simulink model "TEP_Final_NoScript"  (R2024a)
settings: Solver=FixedStepAuto  StartTime=0.0  StopTime=10  FixedStep=1/3600  RelTol=1e-3
model workspace (MAT data in the model file):
  AD : Simulink.Parameter (value not decoded)
  AG : Simulink.Parameter (value not decoded)
  AH : Simulink.Parameter (value not decoded)
  AV : Simulink.Parameter (value not decoded)
  AVP : Simulink.Parameter (value not decoded)
  BCHL : Simulink.Parameter (value not decoded)
  BCHV : Simulink.Parameter (value not decoded)
  BD : Simulink.Parameter (value not decoded)
  BG : Simulink.Parameter (value not decoded)
  BH : Simulink.Parameter (value not decoded)
  BVP : Simulink.Parameter (value not decoded)
  CD : Simulink.Parameter (value not decoded)
  CG : Simulink.Parameter (value not decoded)
  CH : Simulink.Parameter (value not decoded)
  CVP : Simulink.Parameter (value not decoded)
  XMW : Simulink.Parameter (value not decoded)
  XNS : Simulink.Parameter (value not decoded)
  XNSE : Simulink.Parameter (value not decoded)
symbols that are objects in the model workspace (value not decoded): AD, AG, AH, AV, AVP, BD, BG, BH, BVP, CD, CG, CH, CVP, XMW, XNS, XNSE
undefined symbols (not defined in the file or in its folder): magnitude, msgbox, SETPT, XMEAS, XMV
libraries: mylib x360, dspindex x28
(part 14 of 14)

== system TEP_Final_NoScript/Random number generator1/Stream Measurements SMEAS Gas analysis/If Action Subsystem3/Subsystem/Stream 9/Subsystem/TESUB6 XMNSED ==
  G : Inport
  Process Noise I=1-12 G New : mylib/Process Noise I=1-12 G New  SystemSampleTime=-1  VariantActivationTime=update diagram  AllowFlexibleInterface=on  Latency=0  AutoFrameSizeCalculation=off
      settings: SourceProductName=TEP Library
  XNSED : Constant  Value=0.1
  XMNSED : Outport  VectorParamsAs1DForOutWhenUnconnected=off
  G_NEW : Outport  Port=2  VectorParamsAs1DForOutWhenUnconnected=off
  wires:
  XNSED/1 -> Process Noise I=1-12 G New/1
  Process Noise I=1-12 G New/1 -> XMNSED/1
  G/1 -> Process Noise I=1-12 G New/2
  Process Noise I=1-12 G New/2 -> G_NEW/1

== system TEP_Final_NoScript/Random number generator1/Stream Measurements SMEAS Gas analysis/If Action Subsystem3/Subsystem/Stream 9/Subsystem/TESUB6 XMNSEE ==
  G : Inport
  Process Noise I=1-12 G New : mylib/Process Noise I=1-12 G New  SystemSampleTime=-1  VariantActivationTime=update diagram  AllowFlexibleInterface=on  Latency=0  AutoFrameSizeCalculation=off
      settings: SourceProductName=TEP Library
  XNSEE : Constant  Value=0.25
  XMNSEE : Outport  VectorParamsAs1DForOutWhenUnconnected=off
  G_NEW : Outport  Port=2  VectorParamsAs1DForOutWhenUnconnected=off
  wires:
  XNSEE/1 -> Process Noise I=1-12 G New/1
  Process Noise I=1-12 G New/1 -> XMNSEE/1
  G/1 -> Process Noise I=1-12 G New/2
  Process Noise I=1-12 G New/2 -> G_NEW/1

== system TEP_Final_NoScript/Random number generator1/Stream Measurements SMEAS Gas analysis/If Action Subsystem3/Subsystem/Stream 9/Subsystem/TESUB6 XMNSEF ==
  G : Inport
  Process Noise I=1-12 G New : mylib/Process Noise I=1-12 G New  SystemSampleTime=-1  VariantActivationTime=update diagram  AllowFlexibleInterface=on  Latency=0  AutoFrameSizeCalculation=off
      settings: SourceProductName=TEP Library
  XNSEF : Constant  Value=0.025
  XMNSEF : Outport  VectorParamsAs1DForOutWhenUnconnected=off
  G_NEW : Outport  Port=2  VectorParamsAs1DForOutWhenUnconnected=off
  wires:
  XNSEF/1 -> Process Noise I=1-12 G New/1
  Process Noise I=1-12 G New/1 -> XMNSEF/1
  G/1 -> Process Noise I=1-12 G New/2
  Process Noise I=1-12 G New/2 -> G_NEW/1

== system TEP_Final_NoScript/Random number generator1/Stream Measurements SMEAS Gas analysis/If Action Subsystem3/Subsystem/Stream 9/Subsystem/TESUB6 XMNSEG ==
  G : Inport
  Process Noise I=1-12 G New : mylib/Process Noise I=1-12 G New  SystemSampleTime=-1  VariantActivationTime=update diagram  AllowFlexibleInterface=on  Latency=0  AutoFrameSizeCalculation=off
      settings: SourceProductName=TEP Library
  XNSEG : Constant  Value=0.05
  XMNSEG : Outport  VectorParamsAs1DForOutWhenUnconnected=off
  G_NEW : Outport  Port=2  VectorParamsAs1DForOutWhenUnconnected=off
  wires:
  XNSEG/1 -> Process Noise I=1-12 G New/1
  Process Noise I=1-12 G New/1 -> XMNSEG/1
  G/1 -> Process Noise I=1-12 G New/2
  Process Noise I=1-12 G New/2 -> G_NEW/1

== system TEP_Final_NoScript/Random number generator1/Stream Measurements SMEAS Gas analysis/If Action Subsystem3/Subsystem/Stream 9/Subsystem/TESUB6 XMNSEH ==
  G : Inport
  Process Noise I=1-12 G New : mylib/Process Noise I=1-12 G New  SystemSampleTime=-1  VariantActivationTime=update diagram  AllowFlexibleInterface=on  Latency=0  AutoFrameSizeCalculation=off
      settings: SourceProductName=TEP Library
  XNSEH : Constant  Value=0.05
  XMNSEH : Outport  VectorParamsAs1DForOutWhenUnconnected=off
  G_NEW : Outport  Port=2  VectorParamsAs1DForOutWhenUnconnected=off
  wires:
  XNSEH/1 -> Process Noise I=1-12 G New/1
  Process Noise I=1-12 G New/1 -> XMNSEH/1
  G/1 -> Process Noise I=1-12 G New/2
  Process Noise I=1-12 G New/2 -> G_NEW/1

== system TEP_Final_NoScript/Random number generator1/Stream Measurements SMEAS Product analysis/If Action Subsystem3/Subsystem/Subsystem1/Subsystem/TESUB6 XMNSED ==
  G : Inport
  Process Noise I=1-12 G New : mylib/Process Noise I=1-12 G New  SystemSampleTime=-1  VariantActivationTime=update diagram  AllowFlexibleInterface=on  Latency=0  AutoFrameSizeCalculation=off
      settings: SourceProductName=TEP Library
  XNS(37) : Constant  Value=0.01
  XMNS : Outport  VectorParamsAs1DForOutWhenUnconnected=off
  G_NEW : Outport  Port=2  VectorParamsAs1DForOutWhenUnconnected=off
  wires:
  XNS(37)/1 -> Process Noise I=1-12 G New/1
  Process Noise I=1-12 G New/1 -> XMNS/1
  G/1 -> Process Noise I=1-12 G New/2
  Process Noise I=1-12 G New/2 -> G_NEW/1

== system TEP_Final_NoScript/Random number generator1/Stream Measurements SMEAS Product analysis/If Action Subsystem3/Subsystem/Subsystem1/Subsystem/TESUB6 XMNSEE ==
  G : Inport
  Process Noise I=1-12 G New : mylib/Process Noise I=1-12 G New  SystemSampleTime=-1  VariantActivationTime=update diagram  AllowFlexibleInterface=on  Latency=0  AutoFrameSizeCalculation=off
      settings: SourceProductName=TEP Library
  XNS(38) : Constant  Value=0.01
  XMNS : Outport  VectorParamsAs1DForOutWhenUnconnected=off
  G_NEW : Outport  Port=2  VectorParamsAs1DForOutWhenUnconnected=off
  wires:
  XNS(38)/1 -> Process Noise I=1-12 G New/1
  Process Noise I=1-12 G New/1 -> XMNS/1
  G/1 -> Process Noise I=1-12 G New/2
  Process Noise I=1-12 G New/2 -> G_NEW/1

== system TEP_Final_NoScript/Random number generator1/Stream Measurements SMEAS Product analysis/If Action Subsystem3/Subsystem/Subsystem1/Subsystem/TESUB6 XMNSEF ==
  G : Inport
  Process Noise I=1-12 G New : mylib/Process Noise I=1-12 G New  SystemSampleTime=-1  VariantActivationTime=update diagram  AllowFlexibleInterface=on  Latency=0  AutoFrameSizeCalculation=off
      settings: SourceProductName=TEP Library
  XNS(39) : Constant  Value=0.01
  XMNS : Outport  VectorParamsAs1DForOutWhenUnconnected=off
  G_NEW : Outport  Port=2  VectorParamsAs1DForOutWhenUnconnected=off
  wires:
  XNS(39)/1 -> Process Noise I=1-12 G New/1
  Process Noise I=1-12 G New/1 -> XMNS/1
  G/1 -> Process Noise I=1-12 G New/2
  Process Noise I=1-12 G New/2 -> G_NEW/1

== system TEP_Final_NoScript/Random number generator1/Stream Measurements SMEAS Product analysis/If Action Subsystem3/Subsystem/Subsystem1/Subsystem/TESUB6 XMNSEG ==
  G : Inport
  Process Noise I=1-12 G New : mylib/Process Noise I=1-12 G New  SystemSampleTime=-1  VariantActivationTime=update diagram  AllowFlexibleInterface=on  Latency=0  AutoFrameSizeCalculation=off
      settings: SourceProductName=TEP Library
  XNS(40) : Constant  Value=0.5
  XMNS : Outport  VectorParamsAs1DForOutWhenUnconnected=off
  G_NEW : Outport  Port=2  VectorParamsAs1DForOutWhenUnconnected=off
  wires:
  XNS(40)/1 -> Process Noise I=1-12 G New/1
  Process Noise I=1-12 G New/1 -> XMNS/1
  G/1 -> Process Noise I=1-12 G New/2
  Process Noise I=1-12 G New/2 -> G_NEW/1

== system TEP_Final_NoScript/Random number generator1/Stream Measurements SMEAS Product analysis/If Action Subsystem3/Subsystem/Subsystem1/Subsystem/TESUB6 XMNSEH ==
  G : Inport
  Process Noise I=1-12 G New : mylib/Process Noise I=1-12 G New  SystemSampleTime=-1  VariantActivationTime=update diagram  AllowFlexibleInterface=on  Latency=0  AutoFrameSizeCalculation=off
      settings: SourceProductName=TEP Library
  XNS(41) : Constant  Value=0.5
  XMNS : Outport  VectorParamsAs1DForOutWhenUnconnected=off
  G_NEW : Outport  Port=2  VectorParamsAs1DForOutWhenUnconnected=off
  wires:
  XNS(41)/1 -> Process Noise I=1-12 G New/1
  Process Noise I=1-12 G New/1 -> XMNS/1
  G/1 -> Process Noise I=1-12 G New/2
  Process Noise I=1-12 G New/2 -> G_NEW/1

== system TEP_Final_NoScript/Random number generator1/Stream Measurements SMEAS Product analysis/If Action Subsystem3/Subsystem/Subsystem2/Subsystem/TESUB6 XMNSED ==
  G : Inport
  Process Noise I=1-12 G New : mylib/Process Noise I=1-12 G New  SystemSampleTime=-1  VariantActivationTime=update diagram  AllowFlexibleInterface=on  Latency=0  AutoFrameSizeCalculation=off
      settings: SourceProductName=TEP Library
  XNS(37) : Constant  Value=0.01
  XMNS : Outport  VectorParamsAs1DForOutWhenUnconnected=off
  G_NEW : Outport  Port=2  VectorParamsAs1DForOutWhenUnconnected=off
  wires:
  XNS(37)/1 -> Process Noise I=1-12 G New/1
  Process Noise I=1-12 G New/1 -> XMNS/1
  G/1 -> Process Noise I=1-12 G New/2
  Process Noise I=1-12 G New/2 -> G_NEW/1

== system TEP_Final_NoScript/Random number generator1/Stream Measurements SMEAS Product analysis/If Action Subsystem3/Subsystem/Subsystem2/Subsystem/TESUB6 XMNSEE ==
  G : Inport
  Process Noise I=1-12 G New : mylib/Process Noise I=1-12 G New  SystemSampleTime=-1  VariantActivationTime=update diagram  AllowFlexibleInterface=on  Latency=0  AutoFrameSizeCalculation=off
      settings: SourceProductName=TEP Library
  XNS(38) : Constant  Value=0.01
  XMNS : Outport  VectorParamsAs1DForOutWhenUnconnected=off
  G_NEW : Outport  Port=2  VectorParamsAs1DForOutWhenUnconnected=off
  wires:
  XNS(38)/1 -> Process Noise I=1-12 G New/1
  Process Noise I=1-12 G New/1 -> XMNS/1
  G/1 -> Process Noise I=1-12 G New/2
  Process Noise I=1-12 G New/2 -> G_NEW/1

== system TEP_Final_NoScript/Random number generator1/Stream Measurements SMEAS Product analysis/If Action Subsystem3/Subsystem/Subsystem2/Subsystem/TESUB6 XMNSEF ==
  G : Inport
  Process Noise I=1-12 G New : mylib/Process Noise I=1-12 G New  SystemSampleTime=-1  VariantActivationTime=update diagram  AllowFlexibleInterface=on  Latency=0  AutoFrameSizeCalculation=off
      settings: SourceProductName=TEP Library
  XNS(39) : Constant  Value=0.01
  XMNS : Outport  VectorParamsAs1DForOutWhenUnconnected=off
  G_NEW : Outport  Port=2  VectorParamsAs1DForOutWhenUnconnected=off
  wires:
  XNS(39)/1 -> Process Noise I=1-12 G New/1
  Process Noise I=1-12 G New/1 -> XMNS/1
  G/1 -> Process Noise I=1-12 G New/2
  Process Noise I=1-12 G New/2 -> G_NEW/1

== system TEP_Final_NoScript/Random number generator1/Stream Measurements SMEAS Product analysis/If Action Subsystem3/Subsystem/Subsystem2/Subsystem/TESUB6 XMNSEG ==
  G : Inport
  Process Noise I=1-12 G New : mylib/Process Noise I=1-12 G New  SystemSampleTime=-1  VariantActivationTime=update diagram  AllowFlexibleInterface=on  Latency=0  AutoFrameSizeCalculation=off
      settings: SourceProductName=TEP Library
  XNS(40) : Constant  Value=0.5
  XMNS : Outport  VectorParamsAs1DForOutWhenUnconnected=off
  G_NEW : Outport  Port=2  VectorParamsAs1DForOutWhenUnconnected=off
  wires:
  XNS(40)/1 -> Process Noise I=1-12 G New/1
  Process Noise I=1-12 G New/1 -> XMNS/1
  G/1 -> Process Noise I=1-12 G New/2
  Process Noise I=1-12 G New/2 -> G_NEW/1

== system TEP_Final_NoScript/Random number generator1/Stream Measurements SMEAS Product analysis/If Action Subsystem3/Subsystem/Subsystem2/Subsystem/TESUB6 XMNSEH ==
  G : Inport
  Process Noise I=1-12 G New : mylib/Process Noise I=1-12 G New  SystemSampleTime=-1  VariantActivationTime=update diagram  AllowFlexibleInterface=on  Latency=0  AutoFrameSizeCalculation=off
      settings: SourceProductName=TEP Library
  XNS(41) : Constant  Value=0.5
  XMNS : Outport  VectorParamsAs1DForOutWhenUnconnected=off
  G_NEW : Outport  Port=2  VectorParamsAs1DForOutWhenUnconnected=off
  wires:
  XNS(41)/1 -> Process Noise I=1-12 G New/1
  Process Noise I=1-12 G New/1 -> XMNS/1
  G/1 -> Process Noise I=1-12 G New/2
  Process Noise I=1-12 G New/2 -> G_NEW/1

== system TEP_Final_NoScript/Subsystem/Braatz/ 10/CONTROL 6/P Control/ /Pressure limits ==
  "XMV(6) " : Inport
  XMEAS : Inport  Port=2
  Abs : Abs  SaturateOnIntegerOverflow=off
  Bus Selector : BusSelector  OutputSignals=signal3.XMEAS(13)
  Constant : Constant  Value=100
  Constant1 : Constant  Value=0
  If : If  IfExpression=u1 >= 2950  ElseIfExpressions=u1 <= 2300
  If Action Subsystem : Subsystem  TreatAsAtomicUnit=on
  If Action Subsystem1 : Subsystem  TreatAsAtomicUnit=on
  If Action Subsystem2 : Subsystem  TreatAsAtomicUnit=on
  Merge : Merge  Inputs=3
  Subsystem1 : mylib/Braatz Control/Subsystem1  SystemSampleTime=-1  VariantActivationTime=update diagram  AllowFlexibleInterface=on  Latency=0  AutoFrameSizeCalculation=off
      settings: SourceProductName=TEP Library
  XMV(6) : Outport  VectorParamsAs1DForOutWhenUnconnected=off
  wires:
  If/1 -> If Action Subsystem/Action
  Constant1/1 -> If Action Subsystem1/1(In1)
  Merge/1 -> Abs/1
  If/3 -> If Action Subsystem2/Action
  Constant/1 -> If Action Subsystem/1(In1)
  Bus Selector/1 -> If/1  "<XMEAS(13)>"
  If Action Subsystem2/1(Out1) -> Merge/3
  If Action Subsystem1/1(Out1) -> Merge/2
  XMEAS/1 -> Bus Selector/1
  If/2 -> If Action Subsystem1/Action
  If Action Subsystem/1(Out1) -> Merge/1
  "XMV(6) "/1 -> If Action Subsystem2/1(In1)
  Abs/1 -> Subsystem1/1
  Subsystem1/1 -> XMV(6)/1

== system TEP_Final_NoScript/Subsystem/Braatz/ 10/CONTROL 6/P Control/ /Pressure limits/If Action Subsystem ==
  In1 : Inport
  Action Port : ActionPort  ActionPortLabel=if(u1 >= 2950)
  Out1 : Outport  VectorParamsAs1DForOutWhenUnconnected=off
  wires:
  In1/1 -> Out1/1

== system TEP_Final_NoScript/Subsystem/Braatz/ 10/CONTROL 6/P Control/ /Pressure limits/If Action Subsystem1 ==
  In1 : Inport
  Action Port : ActionPort  ActionPortLabel=elseif(u1 <= 2300)
  Out1 : Outport  VectorParamsAs1DForOutWhenUnconnected=off
  wires:
  In1/1 -> Out1/1

== system TEP_Final_NoScript/Subsystem/Braatz/ 10/CONTROL 6/P Control/ /Pressure limits/If Action Subsystem2 ==
  In1 : Inport
  Action Port : ActionPort  ActionPortLabel=else
  Out1 : Outport  VectorParamsAs1DForOutWhenUnconnected=off
  wires:
  In1/1 -> Out1/1

== matlab function TEP_Final_NoScript/Random number generator1/Stream Measurements SMEAS/MATLAB Function ==
  data: XNSE input; GE output; GE input; ISD input; Time input; XMNSE output
function [GE,XMNSE] = ProcessNoise(XNSE,GE,ISD,Time)

X =zeros(24,1);
RN=zeros(24*12+1,1);
RN(1,1)=GE;
TESUB7 = zeros(12,24);

if Time > 0.0 && ISD == 0

    for I=1:24
        
    TESUB7_value = zeros(1,24);
    
        for It =1:12
    
            RN((12*I-11+It),1) = mod(RN((12*I-11+It-1),1) * 9228907,4294967296);
                if It >= 0
                    TESUB7_value(I) = RN((12*I-11+It),1) / 4294967296;
                else
                    TESUB7_value(I) = 2 * RN((12*I-11+It),1) / 4294967296 - 1;
                end
            TESUB7(It,I)=TESUB7_value(I); 
            X(I) = X(I) + TESUB7(It,I);
        end 
    
        X(I) = (X(I) - 6) * XNSE(I,1);
        XMNSE = X;
    end 
    
    GE = RN(end);
    
else
    XMNSE = zeros(24,1);
    GE = RN(1,1);
end

== matlab function TEP_Final_NoScript/Separator/TCS Initial Temperature in Separator °C /MATLAB Function ==
  data: AH input; TCS output; BH input; CH input; AG input; BG input; CG input; AV input; XMW input; XLS input; ETS input; UTLS input; ITY input; J output; TCS input
function [TCS,J] = TempLoop(AH,BH,CH,AG,BG,CG,AV,XMW,XLS,ETS,UTLS,ITY,TCS)

ESS = ETS/UTLS;
     
Z = XLS;
T = TCS;
H = ESS;
TIN=T;

for J = 1:100
	
	if ITY == 0
    	HTEST = 0;
		for I = 1:8
      		HI = T * (AH(I,1) + BH(I,1) * T / 2 + CH(I,1) * T^2 / 3);
      		HI = 1.8 * HI;
      		HTEST = HTEST + Z(I,1) * XMW(I,1) * HI;
		end
	else
      	HTEST = 0;
		for I = 1:8 
      		HI = T * (AG(I,1) + BG(I,1) * T / 2 + CG(I,1) * T^2 / 3);
      		HI = 1.8 * HI;
      		HI = HI + AV(I,1);
      		HTEST = HTEST + Z(I,1) * XMW(I,1) * HI;
		end
    end
        if ITY == 2
         	R1 = 3.57696 / 1000000;
        	HTEST = HTEST - R1 * (T + 273.15);
    	end
		
    ERR = HTEST - H;
	
	if ITY == 0
      	DH = 0.0;
    	for I = 1:8
      		DHI = AH(I,1) + BH(I,1) * T + CH(I,1) * T^2;
      		DHI = 1.8 * DHI;
      		DH = DH + Z(I,1) * XMW(I,1) * DHI;
		end
	else
      	DH=0.0;
    	for I = 1:8
      		DHI = AG(I,1) + BG(I,1) * T + CG(I,1) * T^2;
      		DHI = 1.8 * DHI;
      		DH = DH + Z(I,1) * XMW(I,1) * DHI;
		end
    end
    
    if ITY == 2
      	R3 = 3.57696/1000000;
     	DH = DH - R3;
 	end
	
    DT = -ERR / DH;
    T = T + DT;
  	if abs(DT) < 1*10^(-12)
    	break
  	end
  	if J == 100
  		T = TIN;
  	end
end
TCS = T;

== matlab function TEP_Final_NoScript/Reactor/TCR Initial Temperature in Reactor °C /MATLAB Function ==
  data: AH input; TCR output; BH input; CH input; AG input; BG input; CG input; AV input; XMW input; XLR input; ETR input; UTLR input; ITY input; TCR input
function TCR  = TempLoop(AH,BH,CH,AG,BG,CG,AV,XMW,XLR,ETR,UTLR,ITY,TCR)

ESR = ETR/UTLR;
     
Z = XLR;
T = TCR;
H = ESR;
TIN=T;

for J = 1:100
	
	if ITY == 0
    	HTEST = 0;
		for I = 1:8
      		HI = T * (AH(I,1) + BH(I,1) * T / 2 + CH(I,1) * T^2 / 3);
      		HI = 1.8 * HI;
      		HTEST = HTEST + Z(I,1) * XMW(I,1) * HI;
		end
	else
      	HTEST = 0;
		for I = 1:8 
      		HI = T * (AG(I,1) + BG(I,1) * T / 2 + CG(I,1) * T^2 / 3);
      		HI = 1.8 * HI;
      		HI = HI + AV(I,1);
      		HTEST = HTEST + Z(I,1) * XMW(I,1) * HI;
		end
    end
        if ITY == 2
         	R1 = 3.57696 / 1000000;
        	HTEST = HTEST - R1 * (T + 273.15);
    	end
		
    ERR = HTEST - H;
	
	if ITY == 0
      	DH = 0.0;
    	for I = 1:8
      		DHI = AH(I,1) + BH(I,1) * T + CH(I,1) * T^2;
      		DHI = 1.8 * DHI;
      		DH = DH + Z(I,1) * XMW(I,1) * DHI;
		end
	else
      	DH=0.0;
    	for I = 1:8
      		DHI = AG(I,1) + BG(I,1) * T + CG(I,1) * T^2;
      		DHI = 1.8 * DHI;
      		DH = DH + Z(I,1) * XMW(I,1) * DHI;
		end
    end
    
    if ITY == 2
      	R3 = 3.57696/1000000;
     	DH = DH - R3;
 	end
	
    DT = -ERR / DH;
    T = T + DT;
  	if abs(DT) < 1*10^(-12)
    	break
  	end
  	if J == 100
  		T = TIN;
  	end
end
TCR = T;

== matlab function TEP_Final_NoScript/Stripper/TCC Initial Temperature in Stripper °C /MATLAB Function ==
  data: AH input; TCC output; BH input; CH input; AG input; BG input; CG input; AV input; XMW input; XLC input; ETC input; UTLC input; ITY input; J output; TCC input
function [TCC,J] = TempLoop(AH,BH,CH,AG,BG,CG,AV,XMW,XLC,ETC,UTLC,ITY,TCC)

ESC = ETC/UTLC;
     
Z = XLC;
T = TCC;
H = ESC;
TIN=T;

for J = 1:100
	
	if ITY == 0
    	HTEST = 0;
		for I = 1:8
      		HI = T * (AH(I,1) + BH(I,1) * T / 2 + CH(I,1) * T^2 / 3);
      		HI = 1.8 * HI;
      		HTEST = HTEST + Z(I,1) * XMW(I,1) * HI;
		end
	else
      	HTEST = 0;
		for I = 1:8 
      		HI = T * (AG(I,1) + BG(I,1) * T / 2 + CG(I,1) * T^2 / 3);
      		HI = 1.8 * HI;
      		HI = HI + AV(I,1);
      		HTEST = HTEST + Z(I,1) * XMW(I,1) * HI;
		end
    end
        if ITY == 2
         	R1 = 3.57696 / 1000000;
        	HTEST = HTEST - R1 * (T + 273.15);
    	end
		
    ERR = HTEST - H;
	
	if ITY == 0
      	DH = 0.0;
    	for I = 1:8
      		DHI = AH(I,1) + BH(I,1) * T + CH(I,1) * T^2;
      		DHI = 1.8 * DHI;
      		DH = DH + Z(I,1) * XMW(I,1) * DHI;
		end
	else
      	DH=0.0;
    	for I = 1:8
      		DHI = AG(I,1) + BG(I,1) * T + CG(I,1) * T^2;
      		DHI = 1.8 * DHI;
      		DH = DH + Z(I,1) * XMW(I,1) * DHI;
		end
    end
    
    if ITY == 2
      	R3 = 3.57696/1000000;
     	DH = DH - R3;
 	end
	
    DT = -ERR / DH;
    T = T + DT;
  	if abs(DT) < 1*10^(-12)
    	break
  	end
  	if J == 100
  		T = TIN;
  	end
end
TCC = T;

== matlab function TEP_Final_NoScript/Mixing Zone/TCV Initial Temperature in Mixing zone °C /MATLAB Function ==
  data: AH input; TCV output; BH input; CH input; AG input; BG input; CG input; AV input; XMW input; XVV input; ETV input; UTVV input; ITY input; J output; TCV input
function [TCV,J] = TempLoop(AH,BH,CH,AG,BG,CG,AV,XMW,XVV,ETV,UTVV,ITY,TCV)

ESV = ETV/UTVV;
     
Z = XVV;
T = TCV;
H = ESV;
TIN=T;

for J = 1:100
	
	if ITY == 0
    	HTEST = 0;
		for I = 1:8
      		HI = T * (AH(I,1) + BH(I,1) * T / 2 + CH(I,1) * T^2 / 3);
      		HI = 1.8 * HI;
      		HTEST = HTEST + Z(I,1) * XMW(I,1) * HI;
		end
	else
      	HTEST = 0;
		for I = 1:8 
      		HI = T * (AG(I,1) + BG(I,1) * T / 2 + CG(I,1) * T^2 / 3);
      		HI = 1.8 * HI;
      		HI = HI + AV(I,1);
      		HTEST = HTEST + Z(I,1) * XMW(I,1) * HI;
		end
    end
        if ITY == 2
         	R1 = 3.57696 / 1000000;
        	HTEST = HTEST - R1 * (T + 273.15);
    	end
		
    ERR = HTEST - H;
	
	if ITY == 0
      	DH = 0.0;
    	for I = 1:8
      		DHI = AH(I,1) + BH(I,1) * T + CH(I,1) * T^2;
      		DHI = 1.8 * DHI;
      		DH = DH + Z(I,1) * XMW(I,1) * DHI;
		end
	else
      	DH=0.0;
    	for I = 1:8
      		DHI = AG(I,1) + BG(I,1) * T + CG(I,1) * T^2;
      		DHI = 1.8 * DHI;
      		DH = DH + Z(I,1) * XMW(I,1) * DHI;
		end
    end
    
    if ITY == 2
      	R3 = 3.57696/1000000;
     	DH = DH - R3;
 	end
	
    DT = -ERR / DH;
    T = T + DT;
  	if abs(DT) < 1*10^(-12)
    	break
  	end
  	if J == 100
  		T = TIN;
  	end
end
TCV = T;

== matlab function TEP_Final_NoScript/Random number generator1/Process Measurements XMEAS(I) I=1-22/MATLAB Function ==
  data: XNS input; G output; G input; ISD input; Time input; XMNS output
function [G,XMNS] = ProcessNoise(XNS,G,ISD,Time)

X =zeros(22,1);
RN=zeros(22*12+1,1);
RN(1,1)=G;
TESUB7 = zeros(12,22);

if Time > 0.0 && ISD == 0

    for I=1:22
        
    TESUB7_value = zeros(1,22);
    
        for It =1:12
    
            RN((12*I-11+It),1) = mod(RN((12*I-11+It-1),1) * 9228907,4294967296);
                if It >= 0
                    TESUB7_value(I) = RN((12*I-11+It),1) / 4294967296;
                else
                    TESUB7_value(I) = 2 * RN((12*I-11+It),1) / 4294967296 - 1;
                end
            TESUB7(It,I)=TESUB7_value(I); 
            X(I) = X(I) + TESUB7(It,I);
        end 
    
        X(I) = (X(I) - 6) * XNS(I,1);
        XMNS = X;
    end 
    
    G = RN(end);
    
else
    XMNS = zeros(22,1);
    G = RN(1,1);
end
